simulink model "ECE141_Project_5"  (R2019b)
settings: Solver=VariableStepAuto  StartTime=0.0  StopTime=100.0  RelTol=1e-3
settings Model: Creator=stephenchu  LastModifiedBy=stephenchu

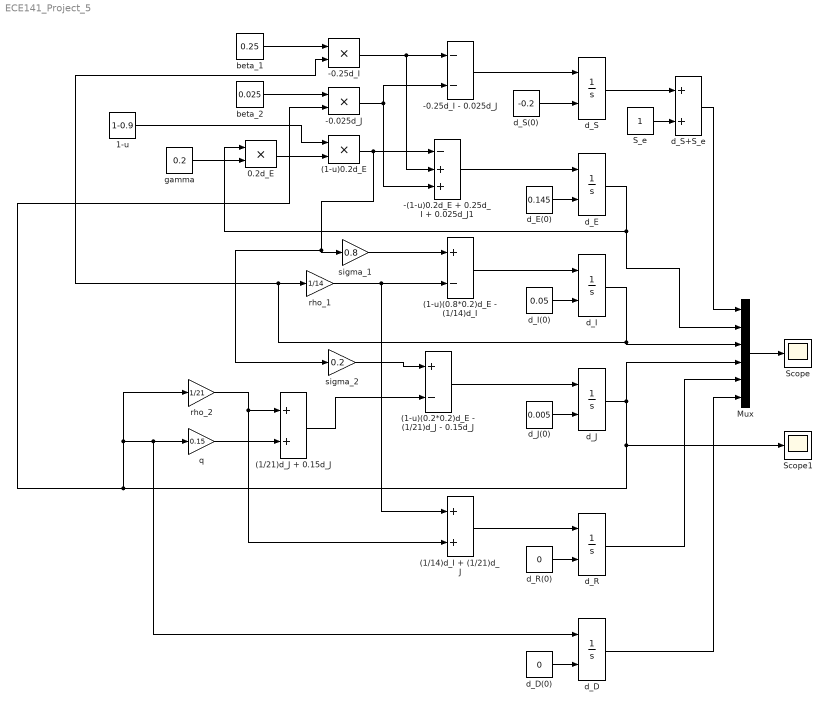
== system ECE141_Project_5 ==
  (1-u)(0.2*0.2)d_E - (1/21)d_J - 0.15d_J : Sum  Inputs=+-
  (1-u)(0.8*0.2)d_E - (1/14)d_I : Sum  Inputs=+-
  (1-u)0.2d_E : Product
  (1/14)d_I + (1/21)d_J : Sum
  (1/21)d_J + 0.15d_J : Sum
  -(1-u)0.2d_E + 0.25d_I + 0.025d_J1 : Sum  Inputs=-++
  -0.025d_J : Product
  -0.25d_I : Product
  -0.25d_I - 0.025d_J : Sum  Inputs=--
  0.2d_E : Product
  1-u : Constant  Value=1-0.9
  Mux : Mux  Inputs=6
  S_e : Constant
  Scope : Scope
  Scope1 : Scope
  beta_1 : Constant  Value=0.25
  beta_2 : Constant  Value=0.025
  d_D : Integrator  InitialConditionSource=external
  d_D(0) : Constant  Value=0
  d_E : Integrator  InitialConditionSource=external
  d_E(0) : Constant  Value=0.145
  d_I : Integrator  InitialConditionSource=external
  d_I(0) : Constant  Value=0.05
  d_J : Integrator  InitialConditionSource=external
  d_J(0) : Constant  Value=0.005
  d_R : Integrator  InitialConditionSource=external
  d_R(0) : Constant  Value=0
  d_S : Integrator  InitialConditionSource=external
  d_S(0) : Constant  Value=-0.2
  d_S+S_e : Sum
  gamma : Constant  Value=0.2
  q : Gain  Gain=0.15
  rho_1 : Gain  Gain=1/14
  rho_2 : Gain  Gain=1/21
  sigma_1 : Gain  Gain=0.8
  sigma_2 : Gain  Gain=0.2
  wires:
  -0.25d_I/1 -> -(1-u)0.2d_E + 0.25d_I + 0.025d_J1/2, -0.25d_I - 0.025d_J/1
  beta_1/1 -> -0.25d_I/1
  beta_2/1 -> -0.025d_J/1
  -0.25d_I - 0.025d_J/1 -> d_S/1
  d_E/1 -> Mux/2, 0.2d_E/1
  -0.025d_J/1 -> -(1-u)0.2d_E + 0.25d_I + 0.025d_J1/3, -0.25d_I - 0.025d_J/2
  -(1-u)0.2d_E + 0.25d_I + 0.025d_J1/1 -> d_E/1
  gamma/1 -> 0.2d_E/2
  0.2d_E/1 -> (1-u)0.2d_E/2
  1-u/1 -> (1-u)0.2d_E/1
  (1-u)0.2d_E/1 -> sigma_1/1, sigma_2/1, -(1-u)0.2d_E + 0.25d_I + 0.025d_J1/1
  sigma_1/1 -> (1-u)(0.8*0.2)d_E - (1/14)d_I/1
  d_I/1 -> Mux/3, rho_1/1, -0.25d_I/2
  rho_1/1 -> (1/14)d_I + (1/21)d_J/1, (1-u)(0.8*0.2)d_E - (1/14)d_I/2
  (1-u)(0.8*0.2)d_E - (1/14)d_I/1 -> d_I/1
  sigma_2/1 -> (1-u)(0.2*0.2)d_E - (1/21)d_J - 0.15d_J/1
  d_J/1 -> Mux/4, Scope1/1, rho_2/1, q/1, d_D/1, -0.025d_J/2
  q/1 -> (1/21)d_J + 0.15d_J/2
  rho_2/1 -> (1/21)d_J + 0.15d_J/1, (1/14)d_I + (1/21)d_J/2
  (1/21)d_J + 0.15d_J/1 -> (1-u)(0.2*0.2)d_E - (1/21)d_J - 0.15d_J/2
  (1-u)(0.2*0.2)d_E - (1/21)d_J - 0.15d_J/1 -> d_J/1
  (1/14)d_I + (1/21)d_J/1 -> d_R/1
  d_S(0)/1 -> d_S/2
  d_E(0)/1 -> d_E/2
  d_J(0)/1 -> d_J/2
  d_R(0)/1 -> d_R/2
  d_D(0)/1 -> d_D/2
  d_R/1 -> Mux/5
  d_D/1 -> Mux/6
  Mux/1 -> Scope/1
  d_I(0)/1 -> d_I/2
  d_S/1 -> d_S+S_e/1
  S_e/1 -> d_S+S_e/2
  d_S+S_e/1 -> Mux/1
